simulink model "lyu_Sim_BEV"  (R2015a)
settings: Solver=ode4  StartTime=0.0  StopTime=0.0  RelTol=1e-3
values from neighbouring files (symbols this model uses):
  g = 9.81    [Uebung1.m]
  m = 10    [Uebung1.m]    (also in Uebung11.m)
undefined symbols (not defined in the file or in its folder): A, alpha, c_alpha, c_W, Cap_Bat, eta_ACDC, eta_DCAC, eta_DCDC, eta_PSM_gen, eta_PSM_mot, f_R, i_diff, J_G, J_H, J_M, J_V, M_cont_gen, M_peak, n_lin, n_max, P_aux, r_dyn, rho, SoC_Start
libraries: simulink x3
settings Model: Creator=Paul  LastModifiedBy=Jason
settings DataIOCC: SignalLoggingSaveFormat=ModelDataLogs
settings OptimizationCC: ExpressionDepthLimit=2147483647  InitFltsAndDblsToZero=on
settings DebuggingCC: SaveWithParameterizedLinksMsg=none  UnderspecifiedInitializationDetection=Classic  MergeDetectMultiDrivingBlocksExec=none  SignalResolutionControl=TryResolveAllWithWarning  SolverPrmCheckMsg=warning  MultiTaskDSMMsg=warning  MultiTaskCondExecSysMsg=none  FcnCallInpInsideContextMsg=EnableAllAsWarning  StateNameClashWarn=warning
settings GRTTargetCC: TargetFcnLib=ansi_tfl_tmw.mat  CombineOutputUpdateFcns=off  GRTInterface=on

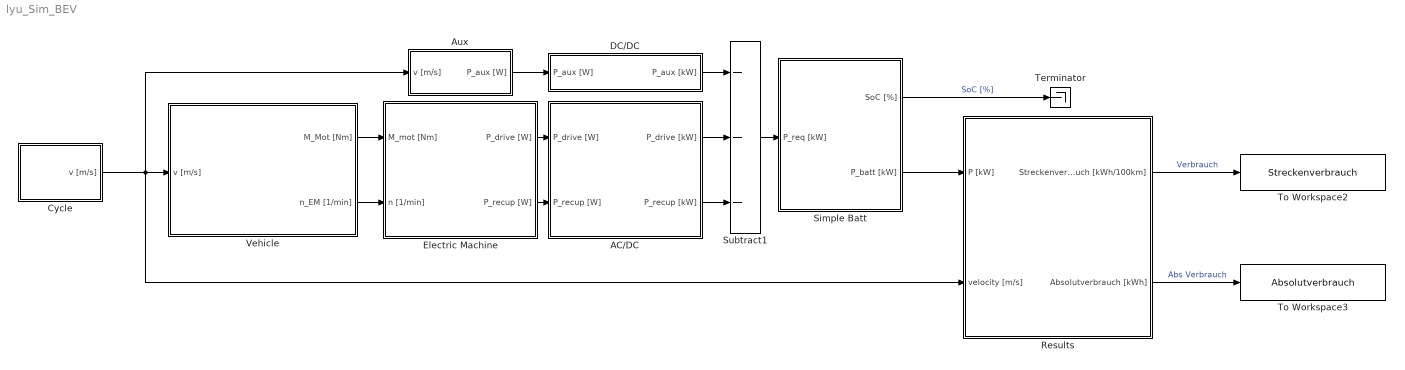
== system lyu_Sim_BEV ==
  AC/DC : Subsystem
  Aux : Subsystem
  Cycle : Subsystem
  DC/DC : Subsystem
  Electric Machine : Subsystem
  Results : Subsystem
  Simple Batt : Subsystem
  Subtract1 : Sum  Inputs=---  InputSameDT=on
  Terminator : Terminator
  To Workspace2 : ToWorkspace  VariableName=Streckenverbrauch  SampleTime=-1
  To Workspace3 : ToWorkspace  VariableName=Absolutverbrauch  SampleTime=-1
  Vehicle : Subsystem
  wires:
  Cycle/1(v [m/s]) -> Aux/1(v [m/s]), Results/2(velocity [m/s]), Vehicle/1(v [m/s])
  DC/DC/1(P_aux [kW]) -> Subtract1/1
  Vehicle/1(M_Mot [Nm]) -> Electric Machine/1(M_mot [Nm])
  Vehicle/2(n_EM [1/min]) -> Electric Machine/2(n [1/min])
  AC/DC/1(P_drive [kW]) -> Subtract1/2
  AC/DC/2(P_recup [kW]) -> Subtract1/3
  Electric Machine/1(P_drive [W]) -> AC/DC/1(P_drive [W])
  Electric Machine/2(P_recup [W]) -> AC/DC/2(P_recup [W])
  Aux/1(P_aux [W]) -> DC/DC/1(P_aux [W])
  Results/2(Absolutverbrauch [kWh]) -> To Workspace3/1  "Abs Verbrauch"
  Subtract1/1 -> Simple Batt/1(P_req [kW])
  Simple Batt/2(P_batt [kW]) -> Results/1(P [kW])
  Results/1(Streckenverbrauch [kWh/100km]) -> To Workspace2/1  "Verbrauch"
  Simple Batt/1(SoC [%]) -> Terminator/1  "SoC [%]"

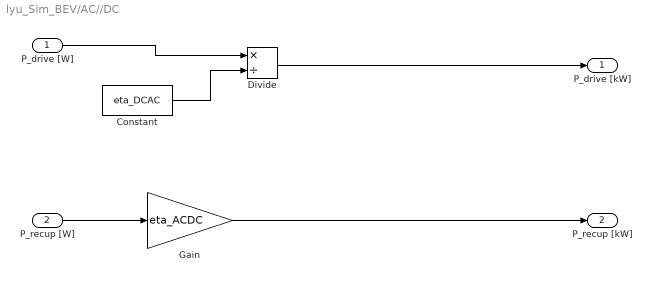
== system lyu_Sim_BEV/AC//DC ==
  P_drive [W] : Inport
  P_recup [W] : Inport  Port=2
  Constant : Constant  Value=eta_DCAC
  Divide : Product  Inputs=*/
  Gain : Gain  Gain=eta_ACDC
  P_drive [kW] : Outport
  P_recup [kW] : Outport  Port=2
  wires:
  P_recup [W]/1 -> Gain/1
  Gain/1 -> P_recup [kW]/1
  P_drive [W]/1 -> Divide/1
  Divide/1 -> P_drive [kW]/1
  Constant/1 -> Divide/2

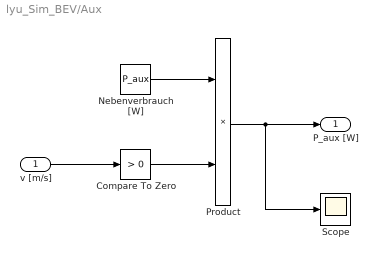
== system lyu_Sim_BEV/Aux ==
  v [m/s] : Inport
  Compare To Zero : simulink/Logic and Bit Operations/Compare To Zero  relop=>  OutDataTypeStr=uint8
  Nebenverbrauch [W] : Constant  Value=P_aux
  Product : Product
  Scope : Scope
      settings: TimeRange=auto  MaxDataPoints=5000  SaveToWorkspace=off  SaveName=ScopeData  YMin=-10  YMax=10  SampleTime=-1
  P_aux [W] : Outport
  wires:
  Product/1 -> Scope/1, P_aux [W]/1
  Nebenverbrauch [W]/1 -> Product/1
  Compare To Zero/1 -> Product/2
  v [m/s]/1 -> Compare To Zero/1

== system lyu_Sim_BEV/Cycle ==
  From Workspace : FromWorkspace  VariableName=velocity  SampleTime=0
  v [m/s] : Outport
  wires:
  From Workspace/1 -> v [m/s]/1

== system lyu_Sim_BEV/DC//DC ==
  P_aux [W] : Inport
  Constant : Constant  Value=eta_DCDC
  Divide : Product  Inputs=*/
  P_aux [kW] : Outport
  wires:
  P_aux [W]/1 -> Divide/1
  Divide/1 -> P_aux [kW]/1
  Constant/1 -> Divide/2

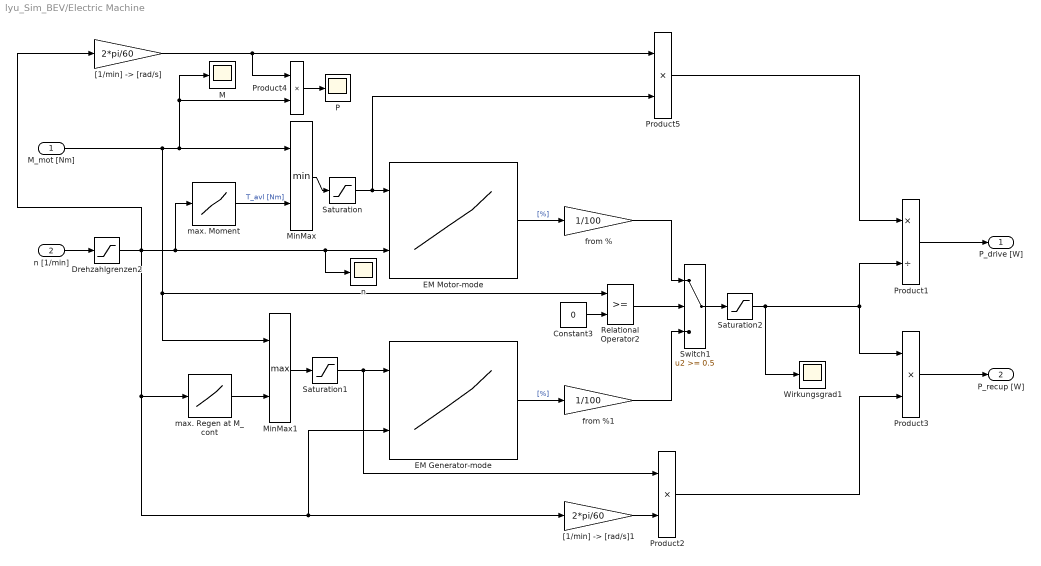
== system lyu_Sim_BEV/Electric Machine ==
  M_mot [Nm] : Inport
  n [1/min] : Inport  Port=2
  Constant3 : Constant  Value=0
  Drehzahlgrenzen2 : Saturate  UpperLimit=n_max  LowerLimit=0
  EM Generator-mode : Lookup2D  RowIndex=M_gen  ColumnIndex=n  Table=eta_PSM_gen
  EM Motor-mode : Lookup2D  RowIndex=M_mot  ColumnIndex=n  Table=eta_PSM_mot
  M : Scope
      settings: TimeRange=auto  MaxDataPoints=5000  SaveName=M_BP  YMin=-10  YMax=10  SampleTime=-1  DataFormat=Array
  MinMax : MinMax  Inputs=2
  MinMax1 : MinMax  Function=max  Inputs=2
  P : Scope
      settings: TimeRange=auto  MaxDataPoints=5000  SaveName=Leistung  YMin=-10  YMax=10  SampleTime=-1  DataFormat=Array
  Product1 : Product  Inputs=*/  RndMeth=Zero
  Product2 : Product  RndMeth=Zero
  Product3 : Product  Inputs=**  RndMeth=Zero
  Product4 : Product  RndMeth=Zero
  Product5 : Product  RndMeth=Zero
  Relational Operator2 : RelationalOperator  OutDataTypeStr=boolean  ZeroCross=off
  Saturation : Saturate  UpperLimit=inf  LowerLimit=0
  Saturation1 : Saturate  UpperLimit=0  LowerLimit=-inf
  Saturation2 : Saturate  UpperLimit=inf  LowerLimit=0.000001
  Switch1 : Switch  Threshold=0.5
  Wirkungsgrad1 : Scope
      settings: TimeRange=auto  MaxDataPoints=5000  SaveName=eta_EM_sim  YMin=-10  YMax=10  SampleTime=-1  DataFormat=Array
  "[1/min] -> [rad/s]" : Gain  Gain=2*pi/60
  "[1/min] -> [rad/s]1" : Gain  Gain=2*pi/60
  from % : Gain  Gain=1/100
  from %1 : Gain  Gain=1/100
  max. Moment : Lookup  InputValues=n_lin  Table=M_peak
  max. Regen at M_cont : Lookup  InputValues=n_lin  Table=M_cont_gen
  n : Scope
      settings: TimeRange=auto  MaxDataPoints=5000  SaveName=n_BP  YMin=-10  YMax=10  SampleTime=-1  DataFormat=Array
  P_drive [W] : Outport
  P_recup [W] : Outport  Port=2
  wires:
  n [1/min]/1 -> Drehzahlgrenzen2/1
  M_mot [Nm]/1 -> MinMax1/1, Relational Operator2/1, M/1, Product4/2, MinMax/1
  "[1/min] -> [rad/s]"/1 -> Product5/1, Product4/1
  Product5/1 -> Product1/1
  MinMax/1 -> Saturation/1
  Drehzahlgrenzen2/1 -> "[1/min] -> [rad/s]"/1, max. Moment/1, EM Motor-mode/2, n/1, EM Generator-mode/2, "[1/min] -> [rad/s]1"/1, max. Regen at M_cont/1
  max. Moment/1 -> MinMax/2  "T_avl [Nm]"
  Saturation/1 -> EM Motor-mode/1, Product5/2
  Relational Operator2/1 -> Switch1/2
  Constant3/1 -> Relational Operator2/2
  Saturation1/1 -> EM Generator-mode/1, Product2/1
  max. Regen at M_cont/1 -> MinMax1/2
  MinMax1/1 -> Saturation1/1
  EM Motor-mode/1 -> from %/1  "[%]"
  EM Generator-mode/1 -> from %1/1  "[%]"
  Switch1/1 -> Saturation2/1
  Saturation2/1 -> Product1/2, Product3/1, Wirkungsgrad1/1
  Product1/1 -> P_drive [W]/1
  from %/1 -> Switch1/1
  from %1/1 -> Switch1/3
  "[1/min] -> [rad/s]1"/1 -> Product2/2
  Product2/1 -> Product3/2
  Product3/1 -> P_recup [W]/1
  Product4/1 -> P/1

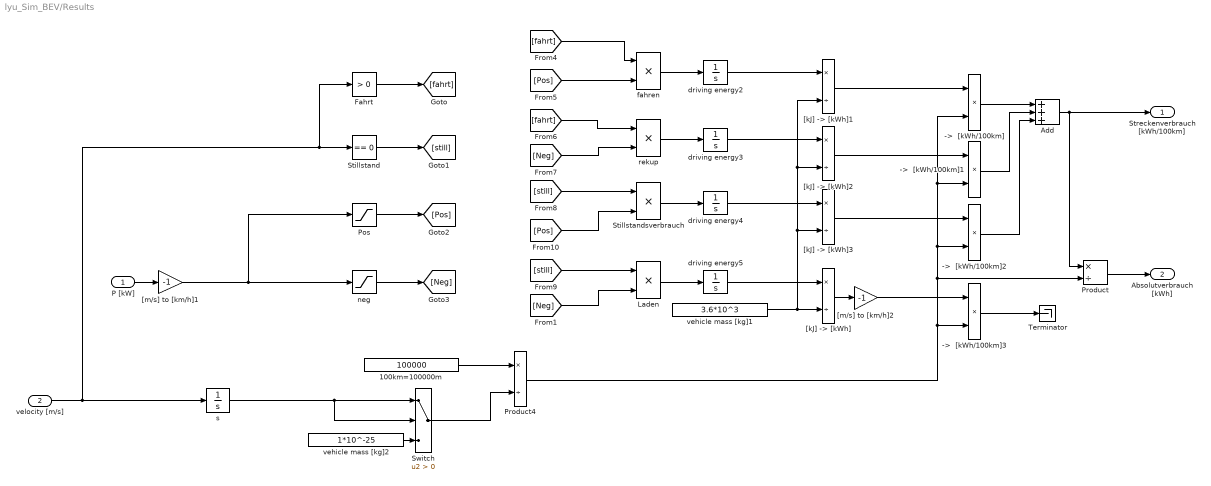
== system lyu_Sim_BEV/Results ==
  P [kW] : Inport
  velocity [m/s] : Inport  Port=2
  ->  [kWh/100km]{,1..3} (4 alike) : Product  Inputs=**
  100km=100000m : Constant  Value=100000
  Add : Sum  Inputs=+++
  Fahrt : simulink/Logic and Bit Operations/Compare To Zero  relop=>  OutDataTypeStr=boolean
  Laden : Product
  Pos : Saturate  UpperLimit=inf  LowerLimit=0
  Product : Product  Inputs=*/
  Product4 : Product  Inputs=*/  SaturateOnIntegerOverflow=on  InputSameDT=on  OutDataTypeStr=Inherit: Same as first input
  Stillstand : simulink/Logic and Bit Operations/Compare To Zero  relop===  OutDataTypeStr=boolean
  Stillstandsverbrauch : Product
  Switch : Switch  Criteria=u2 > Threshold
  Terminator : Terminator
  [kJ] -> [kWh]{,1..3} (4 alike) : Product  Inputs=*/  SaturateOnIntegerOverflow=on  InputSameDT=on  OutDataTypeStr=Inherit: Same as first input
  "[m/s] to [km/h]1" : Gain  Gain=-1
  "[m/s] to [km/h]2" : Gain  Gain=-1
  driving energy{2..5} (4 alike) : Integrator
  fahren : Product
  neg : Saturate  UpperLimit=0  LowerLimit=-inf
  rekup : Product
  s : Integrator
  vehicle mass [kg]1 : Constant  Value=3.6*10^3
  vehicle mass [kg]2 : Constant  Value=1*10^-25
  Streckenverbrauch [kWh/100km] : Outport
  Absolutverbrauch [kWh] : Outport  Port=2
  wires:
  velocity [m/s]/1 -> s/1, Fahrt/1, Stillstand/1
  P [kW]/1 -> "[m/s] to [km/h]1"/1
  "[m/s] to [km/h]1"/1 -> Pos/1, neg/1
  Fahrt/1 -> [fahrt]
  Stillstand/1 -> [still]
  Pos/1 -> [Pos]
  neg/1 -> [Neg]
  [fahrt] -> fahren/1
  [Pos] -> fahren/2
  [Neg] -> rekup/2
  [fahrt] -> rekup/1
  [still] -> Stillstandsverbrauch/1
  [still] -> Laden/1
  [Pos] -> Stillstandsverbrauch/2
  [Neg] -> Laden/2
  fahren/1 -> driving energy2/1
  rekup/1 -> driving energy3/1
  Stillstandsverbrauch/1 -> driving energy4/1
  Laden/1 -> driving energy5/1
  vehicle mass [kg]1/1 -> "[kJ] -> [kWh]1"/2, "[kJ] -> [kWh]2"/2, "[kJ] -> [kWh]3"/2, "[kJ] -> [kWh]"/2
  driving energy5/1 -> "[kJ] -> [kWh]"/1
  driving energy4/1 -> "[kJ] -> [kWh]3"/1
  driving energy3/1 -> "[kJ] -> [kWh]2"/1
  driving energy2/1 -> "[kJ] -> [kWh]1"/1
  100km=100000m/1 -> Product4/1
  Product4/1 -> ->  [kWh/100km]3/2, ->  [kWh/100km]2/2, ->  [kWh/100km]1/2, ->  [kWh/100km]/2, Product/2
  s/1 -> Switch/2, Switch/1
  vehicle mass [kg]2/1 -> Switch/3
  Switch/1 -> Product4/2
  "[kJ] -> [kWh]1"/1 -> ->  [kWh/100km]/1
  "[kJ] -> [kWh]2"/1 -> ->  [kWh/100km]1/1
  "[kJ] -> [kWh]3"/1 -> ->  [kWh/100km]2/1
  "[kJ] -> [kWh]"/1 -> "[m/s] to [km/h]2"/1
  Add/1 -> Product/1, Streckenverbrauch [kWh/100km]/1
  ->  [kWh/100km]/1 -> Add/1
  ->  [kWh/100km]1/1 -> Add/2
  ->  [kWh/100km]2/1 -> Add/3
  Product/1 -> Absolutverbrauch [kWh]/1
  "[m/s] to [km/h]2"/1 -> ->  [kWh/100km]3/1
  ->  [kWh/100km]3/1 -> Terminator/1

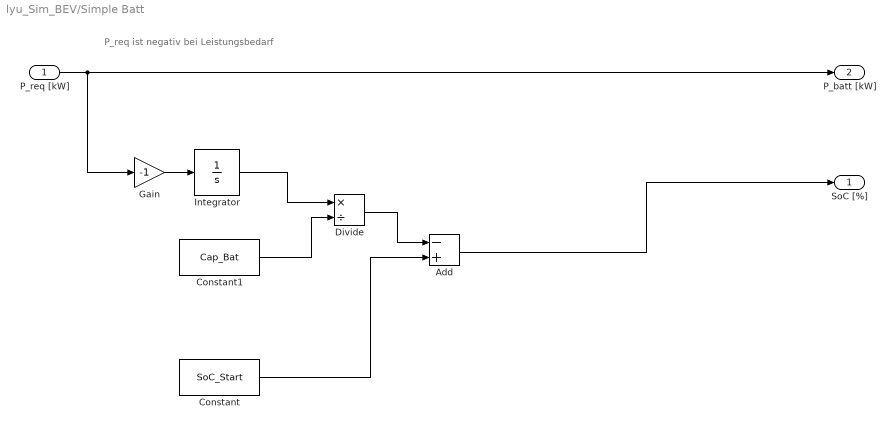
== system lyu_Sim_BEV/Simple Batt ==
  note: P_req ist negativ bei Leistungsbedarf
  P_req [kW] : Inport
  Add : Sum  Inputs=-+
  Constant : Constant  Value=SoC_Start
  Constant1 : Constant  Value=Cap_Bat
  Divide : Product  Inputs=*/
  Gain : Gain  Gain=-1
  Integrator : Integrator
  SoC [%] : Outport
  P_batt [kW] : Outport  Port=2
  wires:
  P_req [kW]/1 -> Gain/1, P_batt [kW]/1
  Add/1 -> SoC [%]/1
  Gain/1 -> Integrator/1
  Integrator/1 -> Divide/1
  Constant1/1 -> Divide/2
  Divide/1 -> Add/1
  Constant/1 -> Add/2

== system lyu_Sim_BEV/Vehicle ==
  v [m/s] : Inport
  Differential : Subsystem
  Resistance : Subsystem
  Wheels : Subsystem
  M_Mot [Nm] : Outport
  n_EM [1/min] : Outport  Port=2
  wires:
  Resistance/1(Fahrwiderstand [N]) -> Wheels/1(F_W_Fzg)
  Resistance/2(v [m/s]1) -> Wheels/2(v [m/s])
  Wheels/1(omega_Rad) -> Differential/1(omega_Rad)
  Wheels/2(M_Diff [Nm]) -> Differential/2("M_Diff [Nm] ")
  Differential/1(n_EM [1/min]) -> n_EM [1/min]/1
  Differential/2(M_mot [Nm]) -> M_Mot [Nm]/1
  v [m/s]/1 -> Resistance/1(v [m/s])

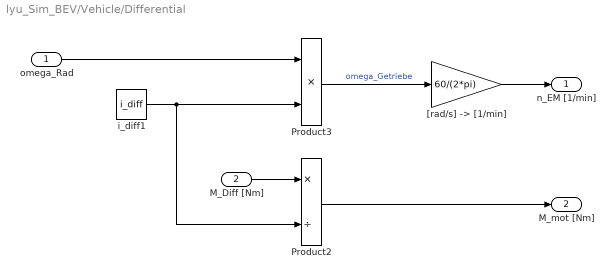
== system lyu_Sim_BEV/Vehicle/Differential ==
  omega_Rad : Inport
  "M_Diff [Nm] " : Inport  Port=2
  Product2 : Product  Inputs=*/  RndMeth=Zero
  Product3 : Product  RndMeth=Zero
  "[rad/s] -> [1/min]" : Gain  Gain=60/(2*pi)
  i_diff1 : Constant  Value=i_diff
  n_EM [1/min] : Outport
  M_mot [Nm] : Outport  Port=2
  wires:
  "M_Diff [Nm] "/1 -> Product2/1
  Product3/1 -> "[rad/s] -> [1/min]"/1  "omega_Getriebe"
  omega_Rad/1 -> Product3/1
  i_diff1/1 -> Product3/2, Product2/2
  Product2/1 -> M_mot [Nm]/1
  "[rad/s] -> [1/min]"/1 -> n_EM [1/min]/1

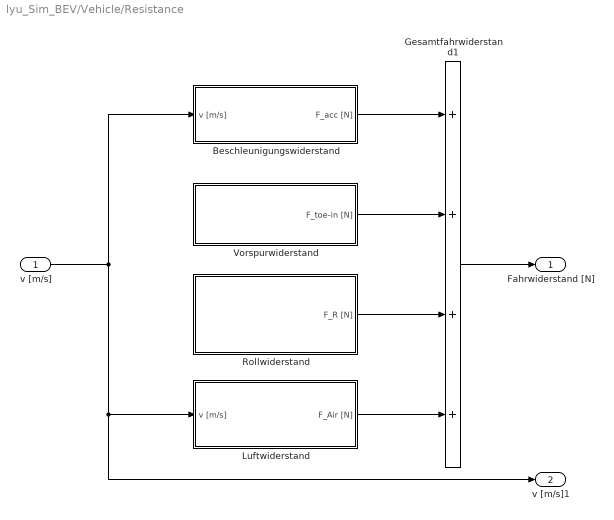
== system lyu_Sim_BEV/Vehicle/Resistance ==
  v [m/s] : Inport
  Beschleunigungswiderstand : Subsystem
  Gesamtfahrwiderstand1 : Sum  Inputs=++++
  Luftwiderstand : Subsystem
  Rollwiderstand : Subsystem
  Vorspurwiderstand : Subsystem
  Fahrwiderstand [N] : Outport
  v [m/s]1 : Outport  Port=2
  wires:
  v [m/s]/1 -> v [m/s]1/1, Luftwiderstand/1(v [m/s]), Beschleunigungswiderstand/1(v [m/s])
  Gesamtfahrwiderstand1/1 -> Fahrwiderstand [N]/1
  Luftwiderstand/1(F_Air [N]) -> Gesamtfahrwiderstand1/4
  Rollwiderstand/1(F_R [N]) -> Gesamtfahrwiderstand1/3
  Vorspurwiderstand/1(F_toe-in [N]) -> Gesamtfahrwiderstand1/2
  Beschleunigungswiderstand/1(F_acc [N]) -> Gesamtfahrwiderstand1/1

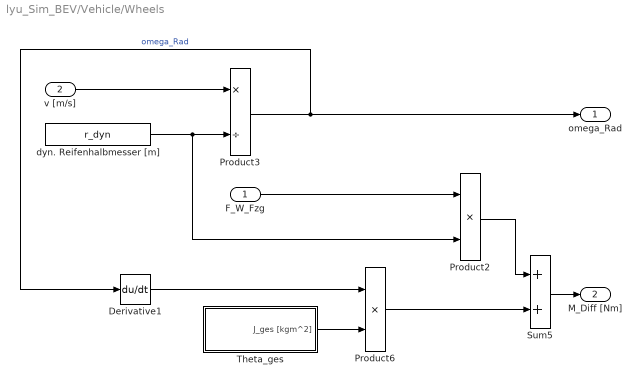
== system lyu_Sim_BEV/Vehicle/Wheels ==
  F_W_Fzg : Inport
  v [m/s] : Inport  Port=2
  Derivative1 : Derivative
  Product2 : Product  RndMeth=Zero
  Product3 : Product  Inputs=*/  RndMeth=Zero
  Product6 : Product  RndMeth=Zero
  Sum5 : Sum
  Theta_ges : Subsystem
  dyn. Reifenhalbmesser [m] : Constant  Value=r_dyn
  omega_Rad : Outport
  M_Diff [Nm] : Outport  Port=2
  wires:
  dyn. Reifenhalbmesser [m]/1 -> Product3/2, Product2/2
  v [m/s]/1 -> Product3/1
  Product3/1 -> Derivative1/1, omega_Rad/1  "omega_Rad"
  F_W_Fzg/1 -> Product2/1
  Product2/1 -> Sum5/1
  Sum5/1 -> M_Diff [Nm]/1
  Derivative1/1 -> Product6/1
  Product6/1 -> Sum5/2
  Theta_ges/1(J_ges [kgm^2]) -> Product6/2

== system lyu_Sim_BEV/Vehicle/Resistance/Beschleunigungswiderstand ==
  v [m/s] : Inport
  Product : Product
  a : Derivative
  "m " : Constant  Value=m
  F_acc [N] : Outport
  wires:
  v [m/s]/1 -> a/1
  Product/1 -> F_acc [N]/1
  a/1 -> Product/1
  "m "/1 -> Product/2

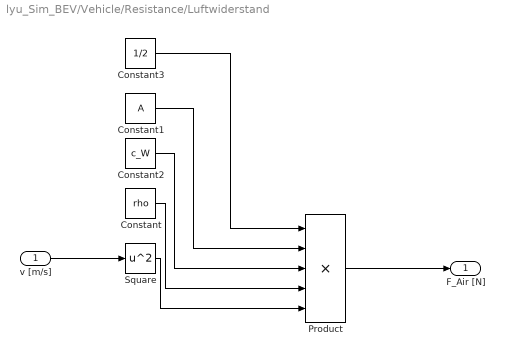
== system lyu_Sim_BEV/Vehicle/Resistance/Luftwiderstand ==
  v [m/s] : Inport
  Constant : Constant  Value=rho
  Constant1 : Constant  Value=A
  Constant2 : Constant  Value=c_W
  Constant3 : Constant  Value=1/2
  Product : Product  Inputs=5
  Square : Math  Operator=square  SaturateOnIntegerOverflow=on
  F_Air [N] : Outport
  wires:
  v [m/s]/1 -> Square/1
  Product/1 -> F_Air [N]/1
  Constant3/1 -> Product/1
  Constant1/1 -> Product/2
  Constant2/1 -> Product/3
  Constant/1 -> Product/4
  Square/1 -> Product/5

== system lyu_Sim_BEV/Vehicle/Resistance/Rollwiderstand ==
  Constant : Constant  Value=f_R
  Constant1 : Constant  Value=m
  Constant2 : Constant  Value=g
  Product : Product  Inputs=3
  F_R [N] : Outport
  wires:
  Product/1 -> F_R [N]/1
  Constant/1 -> Product/1
  Constant1/1 -> Product/2
  Constant2/1 -> Product/3

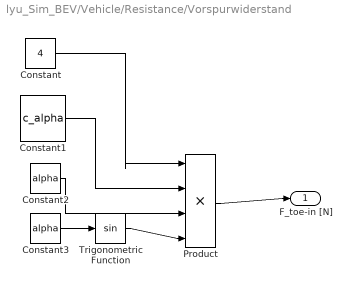
== system lyu_Sim_BEV/Vehicle/Resistance/Vorspurwiderstand ==
  Constant : Constant  Value=4
  Constant1 : Constant  Value=c_alpha
  Constant2 : Constant  Value=alpha
  Constant3 : Constant  Value=alpha
  Product : Product  Inputs=4
  Trigonometric Function : Trigonometry
  F_toe-in [N] : Outport
  wires:
  Product/1 -> F_toe-in [N]/1
  Constant3/1 -> Trigonometric Function/1
  Constant/1 -> Product/1
  Constant1/1 -> Product/2
  Constant2/1 -> Product/3
  Trigonometric Function/1 -> Product/4

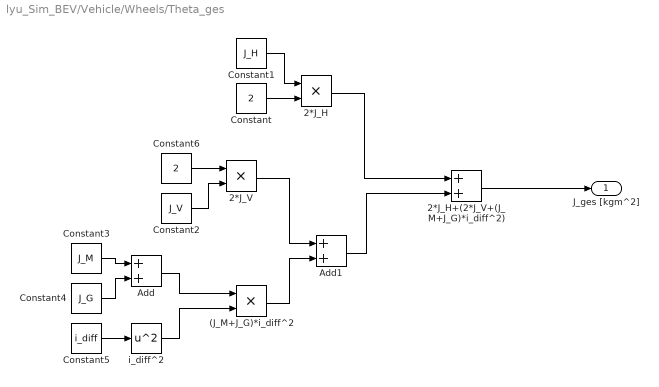
== system lyu_Sim_BEV/Vehicle/Wheels/Theta_ges ==
  (J_M+J_G)*i_diff^2 : Product
  2*J_H : Product
  2*J_H+(2*J_V+(J_M+J_G)*i_diff^2) : Sum
  2*J_V : Product
  Add : Sum
  Add1 : Sum
  Constant : Constant  Value=2
  Constant1 : Constant  Value=J_H
  Constant2 : Constant  Value=J_V
  Constant3 : Constant  Value=J_M
  Constant4 : Constant  Value=J_G
  Constant5 : Constant  Value=i_diff
  Constant6 : Constant  Value=2
  i_diff^2 : Math  Operator=square  SaturateOnIntegerOverflow=on
  J_ges [kgm^2] : Outport
  wires:
  2*J_H+(2*J_V+(J_M+J_G)*i_diff^2)/1 -> J_ges [kgm^2]/1
  Constant5/1 -> i_diff^2/1
  Constant3/1 -> Add/1
  Constant4/1 -> Add/2
  Add/1 -> (J_M+J_G)*i_diff^2/1
  i_diff^2/1 -> (J_M+J_G)*i_diff^2/2
  Constant1/1 -> 2*J_H/1
  Constant/1 -> 2*J_H/2
  Constant6/1 -> 2*J_V/1
  Constant2/1 -> 2*J_V/2
  2*J_V/1 -> Add1/1
  (J_M+J_G)*i_diff^2/1 -> Add1/2
  2*J_H/1 -> 2*J_H+(2*J_V+(J_M+J_G)*i_diff^2)/1
  Add1/1 -> 2*J_H+(2*J_V+(J_M+J_G)*i_diff^2)/2
